simulink model "ACC"  (R2020a)
settings: Solver=ode23t  StartTime=0.0  StopTime=150  MaxStep=0.01  RelTol=1e-3
values from neighbouring files (symbols this model uses):
  ddefault = 5    [a_cruise_control.m]
  K = 0.07536    [a_cruise_control.m]
  rw = 0.3    [a_cruise_control.m]
  tlag = 3    [a_cruise_control.m]
undefined symbols (not defined in the file or in its folder): sigbuilder_block
libraries: simulink x7, dspsigops x1
settings Model: Creator=pruth  LastModifiedBy=pruth

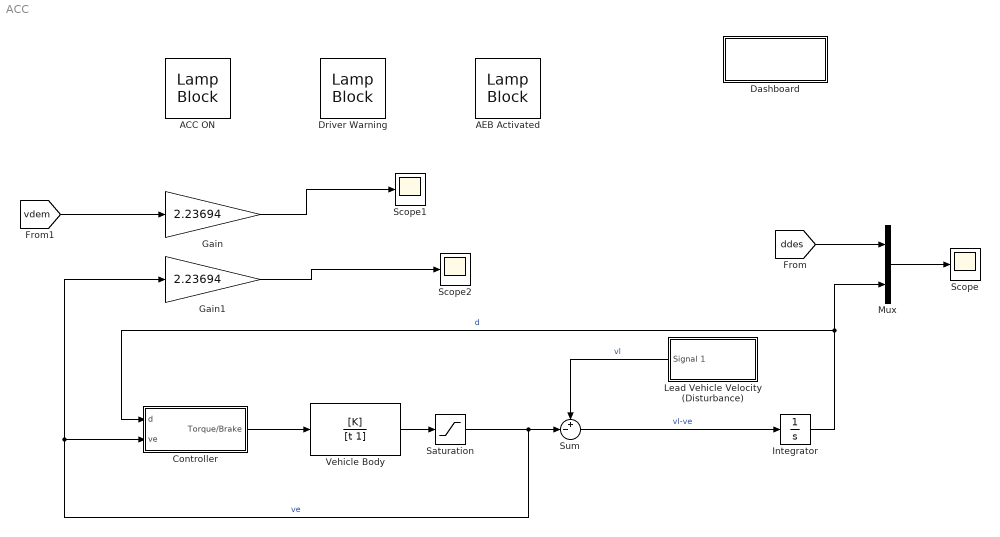
== system ACC ==
  "ACC ON " : LampBlock
  AEB Activated : LampBlock
  Controller : Subsystem
  Dashboard : Subsystem
  Driver Warning : LampBlock
  Gain : Gain  Gain=2.23694
  Gain1 : Gain  Gain=2.23694
  Integrator : Integrator  InitialCondition=100
  Lead Vehicle Velocity (Disturbance) : Subsystem  Tag=STV Subsys  LoadFcn=sigbuilder_block('load');  StartFcn=sigbuilder_block('start');  StopFcn=sigbuilder_block('stop');  ClipboardFcn=sigbuilder_block('clipboard');  mask(Sigbuilder block){tuvar=[0:10]}
      mask help: Simulink:masks:SigbuilderBlock_MD
      mask init:
      | if ~strcmp(get_param(bdroot(gcbh),'SimulationStatus'),'stopped') tuvar = sigbuilder_block('maskInit'); end
      settings: CopyFcn=sigbuilder_block('copy');  DeleteFcn=sigbuilder_block('delete');  ModelCloseFcn=sigbuilder_block('modelClose');  PreSaveFcn=sigbuilder_block('preSave');  PauseFcn=sigbuilder_block('pause');  ContinueFcn=sigbuilder_block('continue');  NameChangeFcn=sigbuilder_block('namechange');  OpenFcn=sigbuilder_block('open',[455.4 76.2 550.8 400.2 ]);  CloseFcn=sigbuilder_block('close');
      mask Display: plot(0, 0, 100, 100,[2, 2, 32, 32, 2], [68, 8, 8, 68, 68],[32, 2], [38, 38], [32, 19, 2],[53, 60, 44], [32, 17, 17, 2],[16, 16, 31, 31]);txt = getActiveGroup(gcbh);text(2, 100, txt,'verticalAlignment', 'top');
  Mux : Mux  Inputs=2
  Saturation : Saturate
  Scope : Scope
  Scope1 : Scope
  Scope2 : Scope
  Sum : Sum  Inputs=+-|
  Vehicle Body : TransferFcn  Numerator=[K]  Denominator=[t 1]
  wires:
  Controller/1(Torque/Brake) -> Vehicle Body/1
  Vehicle Body/1 -> Saturation/1
  Saturation/1 -> Controller/2(ve), Gain1/1, Sum/2  "ve"
  Lead Vehicle Velocity (Disturbance)/1(Signal 1) -> Sum/1  "vl"
  Sum/1 -> Integrator/1  "vl-ve"
  Integrator/1 -> Mux/2, Controller/1(d)  "d"
  [ddes] -> Mux/1
  Mux/1 -> Scope/1
  Gain/1 -> Scope1/1
  Gain1/1 -> Scope2/1
  [vdem] -> Gain/1

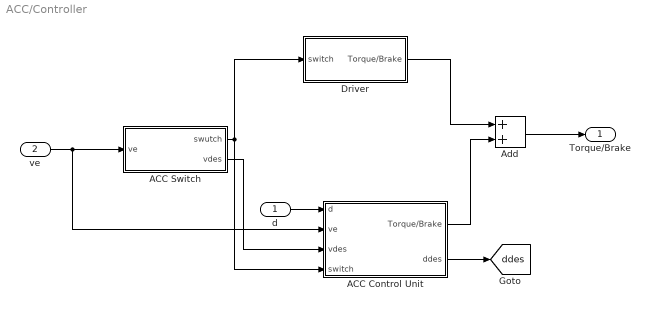
== system ACC/Controller ==
  d : Inport
  ve : Inport  Port=2
  ACC Control Unit : Subsystem
  ACC Switch : Subsystem
  Add : Sum
  Driver : Subsystem
  Torque/Brake : Outport
  tag scope: ddes=global
  wires:
  ve/1 -> ACC Switch/1(ve), ACC Control Unit/2(ve)
  d/1 -> ACC Control Unit/1(d)
  ACC Switch/2(vdes) -> ACC Control Unit/3(vdes)
  ACC Switch/1(swutch) -> Driver/1(switch), ACC Control Unit/4(switch)
  ACC Control Unit/2(ddes) -> [ddes]
  ACC Control Unit/1(Torque/Brake) -> Add/2
  Driver/1(Torque/Brake) -> Add/1
  Add/1 -> Torque/Brake/1

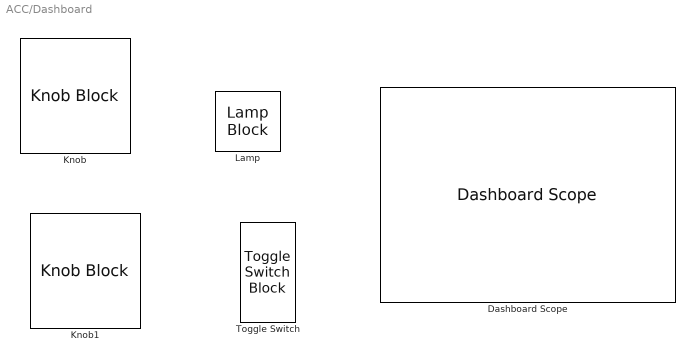
== system ACC/Dashboard ==
  Dashboard Scope : DashboardScope
  Knob : KnobBlock
  Knob1 : KnobBlock
  Lamp : LampBlock
  Toggle Switch : ToggleSwitchBlock
      settings: Values={{'Off', 'On'}, [0 1]}

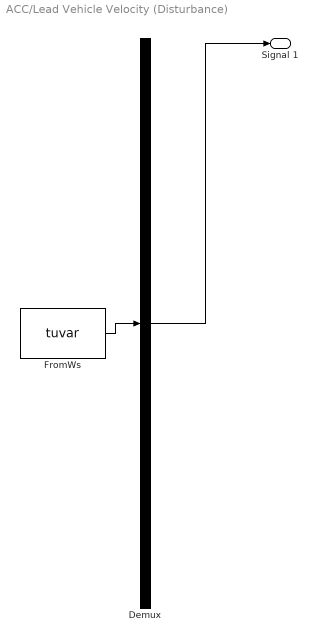
== system ACC/Lead Vehicle Velocity (Disturbance) ==
  Demux : Demux  Tag=STV Demux  Outputs=1
      settings: DisplayOption=none
  FromWs : FromWorkspace  Tag=STV FromWs  VariableName=tuvar
      SigBuilderData=|
      | common.afterFinalStr = 'Extrapolate'
      | common.sampleTime = 0
      | dataSet(1).timeRange = [0 150]
      | dataSet(1).name = 'Scenario1'
      | dataSet(2).timeRange = [0 150]
      | dataSet(2).name = 'Scenario2'
      | dataSet(3).timeRange = [0 150]
      | dataSet(3).name = 'Scenario3'
      | dataSet(4).timeRange = [0 150]
      | dataSet(4).name = 'Scenario4'
      | sbobj.Groups(1).Name = 'Scenario1'
      | sbobj.Groups(1).Signals.Name = 'Signal 1'
      | sbobj.Groups(1).Signals.XData = [0 150]
      | sbobj.Groups(1).Signals.YData = [40 40]
      | sbobj.Groups(1).TimeRange = [0 150]
      | sbobj.Groups(2).Name = 'Scenario2'
      | sbobj.Groups(2).Signals.Name = 'Signal 1'
      | sbobj.Groups(2).Signals.XData = [0 30 70 80 100 150]
      | sbobj.Groups(2).Signals.YData = [25 25 15 15 30 30]
      | sbobj.Groups(2).TimeRange = [0 150]
      | sbobj.Groups(3).Name = 'Scenario3'
      | sbobj.Groups(3).Signals.Name = 'Signal 1'
      | sbobj.Groups(3).Signals.XData = [0 30 70 80 100 150]
      | sbobj.Groups(3).Signals.YData = [25 25 15 15 25 25]
      | sbobj.Groups(3).TimeRange = [0 150]
      | sbobj.Groups(4).Name = 'Scenario4'
      | sbobj.Groups(4).Signals.Name = 'Signal 1'
      | sbobj.Groups(4).Signals.XData = [0 30 70 80 100 150]
      | sbobj.Groups(4).Signals.YData = [25 25 0 0 25 25]
      | sbobj.Groups(4).TimeRange = [0 150]
  Signal 1 : Outport  Tag=STV Outport
  wires:
  Demux/1 -> Signal 1/1
  FromWs/1 -> Demux/1

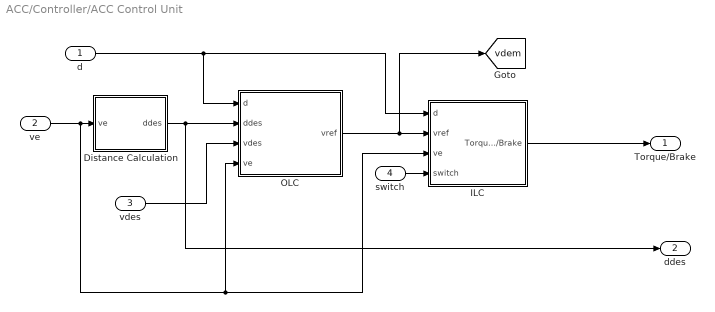
== system ACC/Controller/ACC Control Unit ==
  d : Inport
  ve : Inport  Port=2
  vdes : Inport  Port=3
  switch : Inport  Port=4
  Distance Calculation : Subsystem
  ILC : Subsystem
  OLC : Subsystem
  Torque/Brake : Outport
  ddes : Outport  Port=2
  tag scope: vdem=global
  wires:
  ve/1 -> OLC/4(ve), ILC/3(ve), Distance Calculation/1(ve)
  Distance Calculation/1(ddes) -> OLC/2(ddes), ddes/1
  OLC/1(vref) -> ILC/2(vref), [vdem]
  vdes/1 -> OLC/3(vdes)
  d/1 -> OLC/1(d), ILC/1(d)
  switch/1 -> ILC/4(switch)
  ILC/1(Torque/Brake) -> Torque/Brake/1

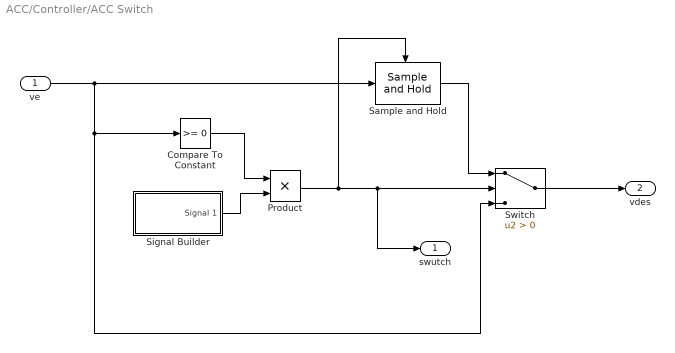
== system ACC/Controller/ACC Switch ==
  ve : Inport
  Compare To Constant : simulink/Logic and Bit Operations/Compare To Constant  relop=>=  const=0  OutDataTypeStr=boolean
  Product : Product
  Sample and Hold : dspsigops/Sample and Hold  trig=Rising edge  initCond=0  latchinput=off
  Signal Builder : Subsystem  Tag=STV Subsys  LoadFcn=sigbuilder_block('load');  StartFcn=sigbuilder_block('start');  StopFcn=sigbuilder_block('stop');  ClipboardFcn=sigbuilder_block('clipboard');  mask(Sigbuilder block){tuvar=[0:10]}
      mask help: Simulink:masks:SigbuilderBlock_MD
      mask init:
      | if ~strcmp(get_param(bdroot(gcbh),'SimulationStatus'),'stopped') tuvar = sigbuilder_block('maskInit'); end
      settings: CopyFcn=sigbuilder_block('copy');  DeleteFcn=sigbuilder_block('delete');  ModelCloseFcn=sigbuilder_block('modelClose');  PreSaveFcn=sigbuilder_block('preSave');  PauseFcn=sigbuilder_block('pause');  ContinueFcn=sigbuilder_block('continue');  NameChangeFcn=sigbuilder_block('namechange');  OpenFcn=sigbuilder_block('open',[194.4 16.8 550.8 400.2 ]);  CloseFcn=sigbuilder_block('close');
      mask Display: plot(0, 0, 100, 100,[2, 2, 32, 32, 2], [68, 8, 8, 68, 68],[32, 2], [38, 38], [32, 19, 2],[53, 60, 44], [32, 17, 17, 2],[16, 16, 31, 31]);txt = getActiveGroup(gcbh);text(2, 100, txt,'verticalAlignment', 'top');
  Switch : Switch  Criteria=u2 > Threshold
  swutch : Outport
  vdes : Outport  Port=2
  wires:
  ve/1 -> Sample and Hold/1, Compare To Constant/1, Switch/3
  Signal Builder/1(Signal 1) -> Product/2
  Compare To Constant/1 -> Product/1
  Product/1 -> swutch/1, Switch/2, Sample and Hold/Trigger
  Switch/1 -> vdes/1
  Sample and Hold/1 -> Switch/1

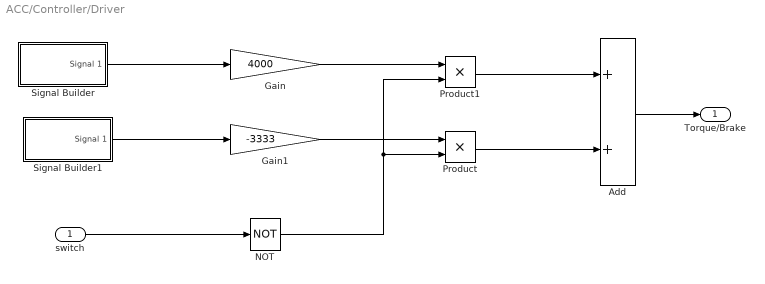
== system ACC/Controller/Driver ==
  switch : Inport
  Add : Sum
  Gain : Gain  Gain=4000
  Gain1 : Gain  Gain=-3333
  NOT : Logic  Operator=NOT  IconShape=distinctive  AllPortsSameDT=off  OutDataTypeStr=boolean
  Product : Product
  Product1 : Product
  Signal Builder : Subsystem  Tag=STV Subsys  LoadFcn=sigbuilder_block('load');  StartFcn=sigbuilder_block('start');  StopFcn=sigbuilder_block('stop');  ClipboardFcn=sigbuilder_block('clipboard');  mask(Sigbuilder block){tuvar=[0:10]}
      mask help: Simulink:masks:SigbuilderBlock_MD
      mask init:
      | if ~strcmp(get_param(bdroot(gcbh),'SimulationStatus'),'stopped') tuvar = sigbuilder_block('maskInit'); end
      settings: CopyFcn=sigbuilder_block('copy');  DeleteFcn=sigbuilder_block('delete');  ModelCloseFcn=sigbuilder_block('modelClose');  PreSaveFcn=sigbuilder_block('preSave');  PauseFcn=sigbuilder_block('pause');  ContinueFcn=sigbuilder_block('continue');  NameChangeFcn=sigbuilder_block('namechange');  OpenFcn=sigbuilder_block('open',[532.2 180.6 449.4 307.2 ]);  CloseFcn=sigbuilder_block('close');
      mask Display: plot(0, 0, 100, 100,[2, 2, 32, 32, 2], [68, 8, 8, 68, 68],[32, 2], [38, 38], [32, 19, 2],[53, 60, 44], [32, 17, 17, 2],[16, 16, 31, 31]);txt = getActiveGroup(gcbh);text(2, 100, txt,'verticalAlignment', 'top');
  Signal Builder1 : Subsystem  Tag=STV Subsys  LoadFcn=sigbuilder_block('load');  StartFcn=sigbuilder_block('start');  StopFcn=sigbuilder_block('stop');  ClipboardFcn=sigbuilder_block('clipboard');  mask(Sigbuilder block){tuvar=[0:10]}
      mask help: Simulink:masks:SigbuilderBlock_MD
      mask init:
      | if ~strcmp(get_param(bdroot(gcbh),'SimulationStatus'),'stopped') tuvar = sigbuilder_block('maskInit'); end
      settings: CopyFcn=sigbuilder_block('copy');  DeleteFcn=sigbuilder_block('delete');  ModelCloseFcn=sigbuilder_block('modelClose');  PreSaveFcn=sigbuilder_block('preSave');  PauseFcn=sigbuilder_block('pause');  ContinueFcn=sigbuilder_block('continue');  NameChangeFcn=sigbuilder_block('namechange');  OpenFcn=sigbuilder_block('open',[657 42 474.6 395.4 ]);  CloseFcn=sigbuilder_block('close');
      mask Display: plot(0, 0, 100, 100,[2, 2, 32, 32, 2], [68, 8, 8, 68, 68],[32, 2], [38, 38], [32, 19, 2],[53, 60, 44], [32, 17, 17, 2],[16, 16, 31, 31]);txt = getActiveGroup(gcbh);text(2, 100, txt,'verticalAlignment', 'top');
  Torque/Brake : Outport
  wires:
  Signal Builder/1(Signal 1) -> Gain/1
  Signal Builder1/1(Signal 1) -> Gain1/1
  switch/1 -> NOT/1
  NOT/1 -> Product/2, Product1/2
  Gain/1 -> Product1/1
  Gain1/1 -> Product/1
  Product/1 -> Add/2
  Product1/1 -> Add/1
  Add/1 -> Torque/Brake/1

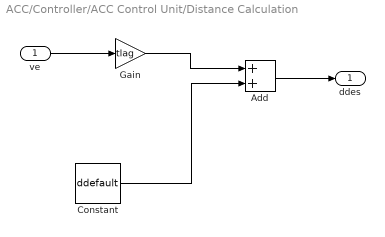
== system ACC/Controller/ACC Control Unit/Distance Calculation ==
  ve : Inport
  Add : Sum
  Constant : Constant  Value=ddefault
  Gain : Gain  Gain=tlag
  ddes : Outport
  wires:
  ve/1 -> Gain/1
  Gain/1 -> Add/1
  Constant/1 -> Add/2
  Add/1 -> ddes/1

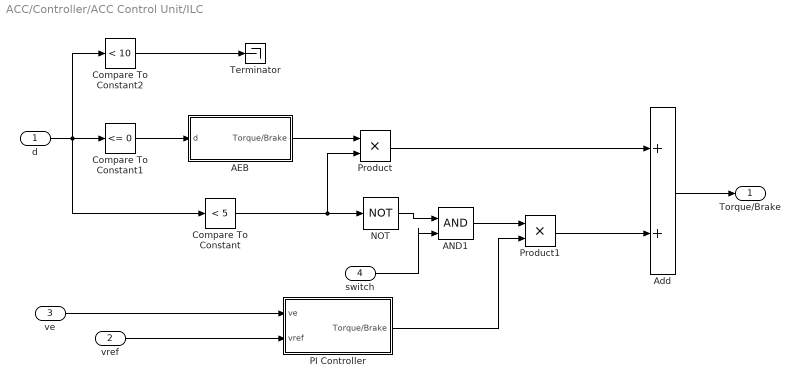
== system ACC/Controller/ACC Control Unit/ILC ==
  d : Inport
  vref : Inport  Port=2
  ve : Inport  Port=3
  switch : Inport  Port=4
  AEB : Subsystem
  AND1 : Logic  IconShape=distinctive  AllPortsSameDT=off  OutDataTypeStr=boolean
  Add : Sum
  Compare To Constant : simulink/Logic and Bit Operations/Compare To Constant  relop=<  const=5  OutDataTypeStr=boolean
  Compare To Constant1 : simulink/Logic and Bit Operations/Compare To Constant  relop=<=  const=0  OutDataTypeStr=boolean
  Compare To Constant2 : simulink/Logic and Bit Operations/Compare To Constant  relop=<  const=10  OutDataTypeStr=boolean
  NOT : Logic  Operator=NOT  IconShape=distinctive  AllPortsSameDT=off  OutDataTypeStr=boolean
  PI Controller : Subsystem
  Product : Product
  Product1 : Product
  Terminator : Terminator
  Torque/Brake : Outport
  wires:
  d/1 -> Compare To Constant2/1, Compare To Constant1/1, Compare To Constant/1
  vref/1 -> PI Controller/2(vref)
  ve/1 -> PI Controller/1(ve)
  Compare To Constant2/1 -> Terminator/1
  Compare To Constant1/1 -> AEB/1(d)
  Compare To Constant/1 -> NOT/1, Product/2
  AEB/1(Torque/Brake) -> Product/1
  NOT/1 -> AND1/1
  switch/1 -> AND1/2
  AND1/1 -> Product1/1
  PI Controller/1(Torque/Brake) -> Product1/2
  Product1/1 -> Add/2
  Product/1 -> Add/1
  Add/1 -> Torque/Brake/1

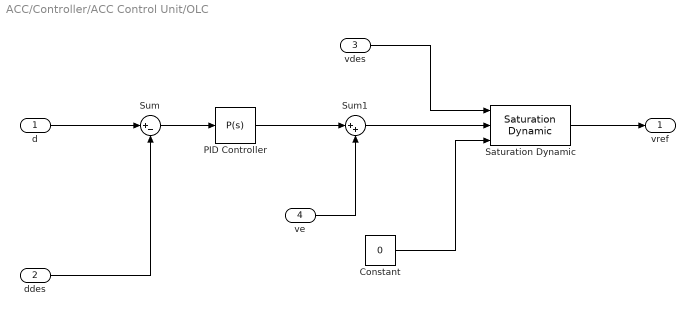
== system ACC/Controller/ACC Control Unit/OLC ==
  d : Inport
  ddes : Inport  Port=2
  vdes : Inport  Port=3
  ve : Inport  Port=4
  Constant : Constant  Value=0
  PID Controller : simulink/Continuous/PID Controller  Controller=P  Form=Parallel  TimeDomain=Continuous-time  UseExternalTs=off  SampleTime=-1  IntegratorMethod=Forward Euler  FilterMethod=Forward Euler  ControllerParametersSource=internal  P=5  I=1  D=0  UseFilter=on  N=100  TunerSelectOption=Transfer Function Based (PID Tuner App)  InitialConditionSource=internal  InitialConditionForIntegrator=0  InitialConditionForFilter=0  DifferentiatorICPrevScaledInput=0  ExternalReset=none  TrackingMode=off  Kt=1  LimitOutput=off  UpperSaturationLimit=inf  LowerSaturationLimit=-inf  LinearizeAsGain=on  AntiWindupMode=none  Kb=1  POutMin=[]  POutMax=[]  IOutMin=[]  IOutMax=[]  DOutMin=[]  DOutMax=[]  NOutMin=[]  NOutMax=[]  SumOutMin=[]  SumOutMax=[]  SaturationOutMin=[]  SaturationOutMax=[]  PParamMin=[]  PParamMax=[]  IParamMin=[]  IParamMax=[]  DParamMin=[]  DParamMax=[]  NParamMin=[]  NParamMax=[]  KbParamMin=[]  KbParamMax=[]  KtParamMin=[]  KtParamMax=[]  KbOutMin=[]  KbOutMax=[]  KtOutMin=[]  KtOutMax=[]  IntegratorOutMin=[]  IntegratorOutMax=[]  FilterOutMin=[]  FilterOutMax=[]  SumI1OutMin=[]  SumI1OutMax=[]  SumI2OutMin=[]  SumI2OutMax=[]  SumI3OutMin=[]  SumI3OutMax=[]  SumI4OutMin=[]  SumI4OutMax=[]  SumDOutMin=[]  SumDOutMax=[]  DifferentiatorOutMin=[]  DifferentiatorOutMax=[]  FilterDiffOutCoefMin=[]  FilterDiffOutCoefMax=[]  ReciprocalOutMin=[]  ReciprocalOutMax=[]  SumDenOutMin=[]  SumDenOutMax=[]  SumNumOutMin=[]  SumNumOutMax=[]  DivideOutMin=[]  DivideOutMax=[]  UdiffTsProdOutMin=[]  UdiffTsProdOutMax=[]  NTsProdOutMin=[]  NTsProdOutMax=[]  UintegralTsProdOutMin=[]  UintegralTsProdOutMax=[]  UngainTsProdOutMin=[]  UngainTsProdOutMax=[]  IntegratorContinuousStateAttributes=''  IntegratorStateMustResolveToSignalObject=off  IntegratorRTWStateStorageClass=Auto  FilterContinuousStateAttributes=''  FilterStateMustResolveToSignalObject=off  FilterRTWStateStorageClass=Auto  ParallelPVariant=InternalParameters  IdealPVariant=Disabled  IVariant=Disabled  DVariant=Disabled  IntegratorVariant=Disabled  SatVariant=Disabled  AWVariant=Disabled  PCopyVariant=Disabled  TRVariant=Disabled  FdbkBlocksVariant=Forward  IdealPFdbkVariant=Disabled  SatFdbkVariant=Disabled  DerivativeFilterVariant=Disabled  NVariant=Disabled  NCopyVariant=Disabled_SignalSpec  FilterICVariant=Disabled  IntegratorICVariant=Disabled  ExternalResetVariant=Disabled  TRSumVariant=Passthrough  SumFdbkVariant=Disabled  SumVariant=Passthrough_P  TsampFilterVariant=InternalTs  TsampNgainVariant=Passthrough  TsampIntegralVariant=Disabled_SignalSpec
  Saturation Dynamic : simulink/Discontinuities/Saturation Dynamic  OutMin=[]  OutMax=[]  OutDataTypeStr=Inherit: Same as second input  OutDataType=fixdt(1, 16)  OutScaling=2^-10  DoSatur=off
  Sum : Sum  Inputs=|+-
  Sum1 : Sum  Inputs=|++
  vref : Outport
  wires:
  d/1 -> Sum/1
  ddes/1 -> Sum/2
  Sum/1 -> PID Controller/1
  PID Controller/1 -> Sum1/1
  ve/1 -> Sum1/2
  Sum1/1 -> Saturation Dynamic/2
  vdes/1 -> Saturation Dynamic/1
  Constant/1 -> Saturation Dynamic/3
  Saturation Dynamic/1 -> vref/1

== system ACC/Controller/ACC Switch/Signal Builder ==
  Demux : Demux  Tag=STV Demux  Outputs=1
      settings: DisplayOption=none
  FromWs : FromWorkspace  Tag=STV FromWs  VariableName=tuvar
      SigBuilderData=|
      | common.afterFinalStr = 'Extrapolate'
      | common.sampleTime = 0
      | dataSet(1).timeRange = [0 150]
      | dataSet(1).name = 'Scenario1'
      | dataSet(2).timeRange = [0 150]
      | dataSet(2).name = 'Scenario2-4'
      | sbobj.Groups(1).Name = 'Scenario1'
      | sbobj.Groups(1).Signals.Name = 'Signal 1'
      | sbobj.Groups(1).Signals.XData = [0 10 10 80 80 150]
      | sbobj.Groups(1).Signals.YData = [0 0 1 1 0 0]
      | sbobj.Groups(1).TimeRange = [0 150]
      | sbobj.Groups(2).Name = 'Scenario2-4'
      | sbobj.Groups(2).Signals.Name = 'Signal 1'
      | sbobj.Groups(2).Signals.XData = [0 10 10 150]
      | sbobj.Groups(2).Signals.YData = [0 0 1 1]
      | sbobj.Groups(2).TimeRange = [0 150]
  Signal 1 : Outport  Tag=STV Outport
  wires:
  Demux/1 -> Signal 1/1
  FromWs/1 -> Demux/1

== system ACC/Controller/Driver/Signal Builder ==
  Demux : Demux  Tag=STV Demux  Outputs=1
      settings: DisplayOption=none
  FromWs : FromWorkspace  Tag=STV FromWs  VariableName=tuvar
      SigBuilderData=|
      | common.afterFinalStr = 'Extrapolate'
      | common.sampleTime = 0
      | dataSet(1).timeRange = [0 150]
      | dataSet(1).name = 'Scenario1'
      | dataSet(2).timeRange = [0 150]
      | dataSet(2).name = 'Scenario2-4'
      | sbobj.Groups(1).Name = 'Scenario1'
      | sbobj.Groups(1).Signals.Name = 'Signal 1'
      | sbobj.Groups(1).Signals.XData = [0 10 10 100 100 120 120 150]
      | sbobj.Groups(1).Signals.YData = [0.7 0.7 0 0 0.3 0.3 0 0]
      | sbobj.Groups(1).TimeRange = [0 150]
      | sbobj.Groups(2).Name = 'Scenario2-4'
      | sbobj.Groups(2).Signals.Name = 'Signal 1'
      | sbobj.Groups(2).Signals.XData = [0 10 10 100 150]
      | sbobj.Groups(2).Signals.YData = [0.7 0.7 0 0 0]
      | sbobj.Groups(2).TimeRange = [0 150]
  Signal 1 : Outport  Tag=STV Outport
  wires:
  Demux/1 -> Signal 1/1
  FromWs/1 -> Demux/1

== system ACC/Controller/Driver/Signal Builder1 ==
  Demux : Demux  Tag=STV Demux  Outputs=1
      settings: DisplayOption=none
  FromWs : FromWorkspace  Tag=STV FromWs  VariableName=tuvar
      SigBuilderData=|
      | common.afterFinalStr = 'Extrapolate'
      | common.sampleTime = 0
      | dataSet(1).timeRange = [0 150]
      | dataSet(1).name = 'Scenario1'
      | dataSet(2).timeRange = [0 150]
      | dataSet(2).name = 'Scenario2-4'
      | sbobj.Groups(1).Name = 'Scenario1'
      | sbobj.Groups(1).Signals.Name = 'Signal 1'
      | sbobj.Groups(1).Signals.XData = [0 80 80 100 100 120 120 150]
      | sbobj.Groups(1).Signals.YData = [0 0 0.1 0.1 0 0 0.05 0.05]
      | sbobj.Groups(1).TimeRange = [0 150]
      | sbobj.Groups(2).Name = 'Scenario2-4'
      | sbobj.Groups(2).Signals.Name = 'Signal 1'
      | sbobj.Groups(2).Signals.XData = [0 150]
      | sbobj.Groups(2).Signals.YData = [0 0]
      | sbobj.Groups(2).TimeRange = [0 150]
  Signal 1 : Outport  Tag=STV Outport
  wires:
  FromWs/1 -> Demux/1
  Demux/1 -> Signal 1/1

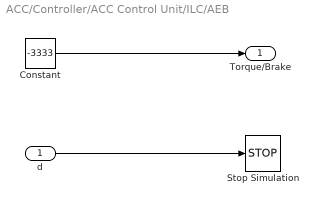
== system ACC/Controller/ACC Control Unit/ILC/AEB ==
  d : Inport
  Constant : Constant  Value=-3333
  Stop Simulation : Stop
  Torque/Brake : Outport
  wires:
  d/1 -> Stop Simulation/1
  Constant/1 -> Torque/Brake/1

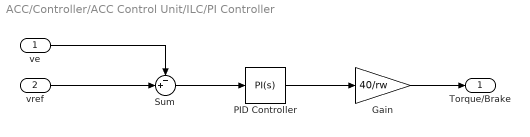
== system ACC/Controller/ACC Control Unit/ILC/PI Controller ==
  ve : Inport
  vref : Inport  Port=2
  Gain : Gain  Gain=40/rw
  PID Controller : simulink/Continuous/PID Controller  Controller=PI  Form=Parallel  TimeDomain=Continuous-time  UseExternalTs=off  SampleTime=-1  IntegratorMethod=Forward Euler  FilterMethod=Forward Euler  ControllerParametersSource=internal  P=10  I=50  D=0  UseFilter=on  N=100  TunerSelectOption=Transfer Function Based (PID Tuner App)  InitialConditionSource=internal  InitialConditionForIntegrator=0  InitialConditionForFilter=0  DifferentiatorICPrevScaledInput=0  ExternalReset=none  TrackingMode=off  Kt=1  LimitOutput=off  UpperSaturationLimit=inf  LowerSaturationLimit=-inf  LinearizeAsGain=on  AntiWindupMode=none  Kb=1  POutMin=[]  POutMax=[]  IOutMin=[]  IOutMax=[]  DOutMin=[]  DOutMax=[]  NOutMin=[]  NOutMax=[]  SumOutMin=[]  SumOutMax=[]  SaturationOutMin=[]  SaturationOutMax=[]  PParamMin=[]  PParamMax=[]  IParamMin=[]  IParamMax=[]  DParamMin=[]  DParamMax=[]  NParamMin=[]  NParamMax=[]  KbParamMin=[]  KbParamMax=[]  KtParamMin=[]  KtParamMax=[]  KbOutMin=[]  KbOutMax=[]  KtOutMin=[]  KtOutMax=[]  IntegratorOutMin=[]  IntegratorOutMax=[]  FilterOutMin=[]  FilterOutMax=[]  SumI1OutMin=[]  SumI1OutMax=[]  SumI2OutMin=[]  SumI2OutMax=[]  SumI3OutMin=[]  SumI3OutMax=[]  SumI4OutMin=[]  SumI4OutMax=[]  SumDOutMin=[]  SumDOutMax=[]  DifferentiatorOutMin=[]  DifferentiatorOutMax=[]  FilterDiffOutCoefMin=[]  FilterDiffOutCoefMax=[]  ReciprocalOutMin=[]  ReciprocalOutMax=[]  SumDenOutMin=[]  SumDenOutMax=[]  SumNumOutMin=[]  SumNumOutMax=[]  DivideOutMin=[]  DivideOutMax=[]  UdiffTsProdOutMin=[]  UdiffTsProdOutMax=[]  NTsProdOutMin=[]  NTsProdOutMax=[]  UintegralTsProdOutMin=[]  UintegralTsProdOutMax=[]  UngainTsProdOutMin=[]  UngainTsProdOutMax=[]  IntegratorContinuousStateAttributes=''  IntegratorStateMustResolveToSignalObject=off  IntegratorRTWStateStorageClass=Auto  FilterContinuousStateAttributes=''  FilterStateMustResolveToSignalObject=off  FilterRTWStateStorageClass=Auto  ParallelPVariant=InternalParameters  IdealPVariant=Disabled  IVariant=InternalParameters  DVariant=Disabled  IntegratorVariant=Continuous  SatVariant=Disabled  AWVariant=Passthrough  PCopyVariant=Disabled  TRVariant=Disabled  FdbkBlocksVariant=Forward  IdealPFdbkVariant=Disabled  SatFdbkVariant=Disabled  DerivativeFilterVariant=Disabled  NVariant=Disabled  NCopyVariant=Disabled_SignalSpec  FilterICVariant=Disabled  IntegratorICVariant=InternalICs  ExternalResetVariant=Disabled  TRSumVariant=Passthrough  SumFdbkVariant=Disabled  SumVariant=Sum_PI  TsampFilterVariant=InternalTs  TsampNgainVariant=Passthrough  TsampIntegralVariant=Passthrough
  Sum : Sum  Inputs=-+|
  Torque/Brake : Outport
  wires:
  vref/1 -> Sum/2
  ve/1 -> Sum/1
  Sum/1 -> PID Controller/1
  PID Controller/1 -> Gain/1
  Gain/1 -> Torque/Brake/1
